simulink model "Acq_HDL"  (R2019b)
settings: Solver=VariableStepAuto  StartTime=0.0  StopTime=time  RelTol=1e-3
values from neighbouring files (symbols this model uses):
  fs = 16367600    [config.m]
  Len = ceil(ms*fs/1000)    [config.m]
libraries: commseqgen3 x4, simulink x3, dsphdlxfrm x2, hdlsllib x2, dspsigops x2, dspswit3 x1, dspsrcs4 x1
settings Model: Creator=nishantmittal  LastModifiedBy=nishantmittal

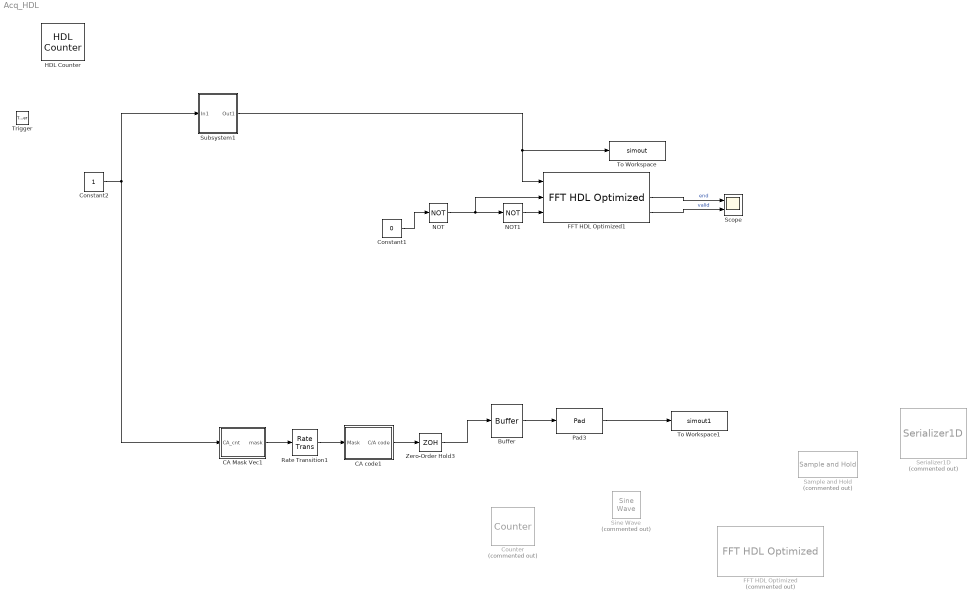
== system Acq_HDL ==
  Trigger : TriggerPort  VariantControl=Variant  PortDimensions=1
  Buffer : Buffer  N=Len  OutputFrames=off
  CA Mask Vec1 : MATLAB Function  TreatAsAtomicUnit=on
  CA code1 : Subsystem
  Constant1 : Constant  Value=0  OutDataTypeStr=Inherit: Inherit via back propagation  SampleTime=-1
  Constant2 : Constant  OutDataTypeStr=Inherit: Inherit via back propagation  SampleTime=-1
  Counter : dspswit3/Counter  Commented=on  Direction=Up  CountEvent=Rising edge  CounterSize=User defined  MaxCount=Len  InitialCount=1  Output=Count and Hit  HitValue=Len  ResetInput=on  SamplesPerFrame=1  Ts=1  CntDtype=single  HitDtype=Logical
  FFT HDL Optimized : dsphdlxfrm/FFT HDL Optimized  Commented=on  FFTLength=2^nextpow2(Len)  Architecture=Streaming Radix 2^2  ComplexMultiplication=Use 4 multipliers and 2 adders  BitReversedOutput=on  BitReversedInput=off  Normalize=off  SimulateUsing=Code generation  RoundingMethod=Floor  ResetInputPort=on  StartOutputPort=off  EndOutputPort=on
      settings: SourceProductName=DSP System Toolbox  SourceProductBaseCode=DS
  FFT HDL Optimized1 : dsphdlxfrm/FFT HDL Optimized  FFTLength=64  Architecture=Streaming Radix 2^2  ComplexMultiplication=Use 4 multipliers and 2 adders  BitReversedOutput=on  BitReversedInput=off  Normalize=off  SimulateUsing=Code generation  RoundingMethod=Floor  ResetInputPort=on  StartOutputPort=off  EndOutputPort=on
      settings: SourceProductName=DSP System Toolbox  SourceProductBaseCode=DS
  HDL Counter : hdlsllib/Sources/HDL Counter  CountType=Count limited  CountInit=0  CountStep=1  CountMax=25  CountFromType=Initial value  CountFrom=0  CountResetPort=off  CountLoadPort=off  CountEnbPort=off  CountDirPort=off  CountDataType=Unsigned  CountWordLen=8  CountFracLen=0  CountSampTime=1
      settings: SourceProductName=Simulink
  NOT : Logic  Operator=NOT  IconShape=distinctive  AllPortsSameDT=off  OutDataTypeStr=boolean
  NOT1 : Logic  Operator=NOT  IconShape=distinctive  AllPortsSameDT=off  OutDataTypeStr=boolean
  Pad3 : dspsigops/Pad  padAlong=Columns  dimsToPad=1  valSrc=Specify via dialog  padVal=0  spec=Output size  padNumOutRowsSpecMethod=Next power of two  numOutRows=1  padNumOutColsSpecMethod=Next power of two  numOutCols=1  isVarDimsMode=off  padBeginning=0  padEnd=0  outSizeMode=User-specified  outSize=1  padSigAt=End  trunc_flag=None  roundingMode=Floor  overflowMode=off  truncOrWrapMode=Truncate  wrap_flag=None
      settings: SourceProductName=DSP System Toolbox  SourceProductBaseCode=DS
  Rate Transition1 : RateTransition  Deterministic=off  OutPortSampleTime=1/(1.023e6)
  Sample and Hold : dspsigops/Sample and Hold  Commented=on  trig=Rising edge  initCond=0  latchinput=on
  Scope : Scope  NumInputPorts=2
  Serializer1D : hdlsllib/HDL Operations/Serializer1D  Commented=on  Ratio=1  IdleCycles=0  validIn=on  startOut=on  validOut=on  inputDataDimensions=-1  inputSampleTime=-1  inputSignalType=auto
      settings: SourceProductName=Simulink  SourceProductBaseCode=SL
  Sine Wave : dspsrcs4/Sine Wave  Commented=on  Amplitude=1  Frequency=100  Phase=0  SampleMode=Discrete  OutComplex=Real  CompMethod=Trigonometric fcn  TableSize=Speed  SampleTime=1/1000  SamplesPerFrame=1  ResetState=Restart at time zero  OutputFrames=off  dataType=single  wordLen=16  udDataType=sfix(16)  fracBitsMode=Best precision  numFracBits=15  OutDataTypeStr=single  LastOutDataTypeStr=single
  Subsystem1 : Subsystem
  To Workspace : ToWorkspace  VariableName=simout  SaveFormat=Timeseries  SampleTime=-1
  To Workspace1 : ToWorkspace  VariableName=simout1  SaveFormat=Timeseries  SampleTime=-1
  Zero-Order Hold3 : ZeroOrderHold  SampleTime=1/fs
  wires:
  Constant1/1 -> NOT/1
  NOT/1 -> FFT HDL Optimized1/2, NOT1/1
  NOT1/1 -> FFT HDL Optimized1/3
  FFT HDL Optimized1/2 -> Scope/1  "end"
  FFT HDL Optimized1/3 -> Scope/2  "valid"
  Zero-Order Hold3/1 -> Buffer/1
  Rate Transition1/1 -> CA code1/1(Mask)
  Constant2/1 -> Subsystem1/1(In1), CA Mask Vec1/1(CA_cnt)
  CA Mask Vec1/1(mask) -> Rate Transition1/1
  CA code1/1(C/A code) -> Zero-Order Hold3/1
  Buffer/1 -> Pad3/1
  Pad3/1 -> To Workspace1/1
  Subsystem1/1(Out1) -> To Workspace/1, FFT HDL Optimized1/1

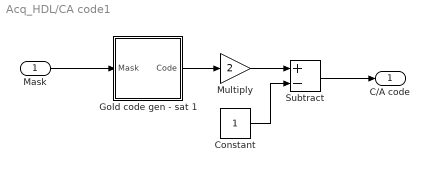
== system Acq_HDL/CA code1 ==
  Mask : Inport
  Constant : Constant
  Gold code gen - sat 1 : Subsystem
  Multiply : Gain  Gain=2
  Subtract : Sum  Inputs=+-
  C/A code : Outport
  wires:
  Subtract/1 -> C/A code/1
  Multiply/1 -> Subtract/1
  Gold code gen - sat 1/1(Code) -> Multiply/1
  Constant/1 -> Subtract/2
  Mask/1 -> Gold code gen - sat 1/1(Mask)

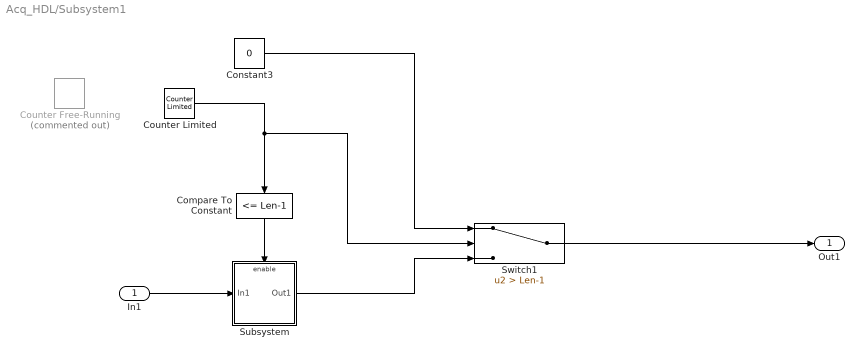
== system Acq_HDL/Subsystem1 ==
  In1 : Inport
  Compare To Constant : simulink/Logic and Bit Operations/Compare To Constant  relop=<=  const=Len-1  OutDataTypeStr=boolean
  Constant3 : Constant  Value=0  OutDataTypeStr=Inherit: Inherit via back propagation  SampleTime=-1
  Counter Free-Running : simulink/Sources/Counter Free-Running  Commented=on  NumBits=3+ nextpow2(Len)  tsamp=-1
  Counter Limited : simulink/Sources/Counter Limited  uplimit=2^nextpow2(Len) - 1  tsamp=-1
  Subsystem : Subsystem
  Switch1 : Switch  Criteria=u2 > Threshold  Threshold=Len-1
  Out1 : Outport
  wires:
  Subsystem/1(Out1) -> Switch1/3
  Switch1/1 -> Out1/1
  In1/1 -> Subsystem/1(In1)
  Compare To Constant/1 -> Subsystem/Enable
  Constant3/1 -> Switch1/1
  Counter Limited/1 -> Switch1/2, Compare To Constant/1

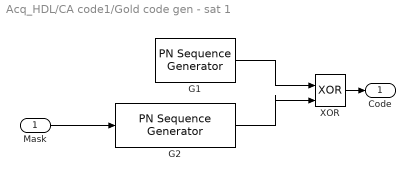
== system Acq_HDL/CA code1/Gold code gen - sat 1 ==
  Mask : Inport
  G1 : commseqgen3/PN Sequence Generator  poly=[10 7 0]  ini_sta=[1 1 1 1 1 1 1 1 1 1]  outBitMaskSource=Dialog parameter  shift=[0 0 0 0 0 0 0 0 0 1]  outVarSiz=off  maxOutSizeMode=Dialog parameter  maxOutSize=[10 1]  Ts=1/(1.023e6)  sampPerFrame=1  reset=off  bitPackedOutputs=off  outDataType=boolean  numPackedBits=8  bitPackDataSigned=off  bitPackedOutDType=double
      settings: SourceProductName=Communications Toolbox
  G2 : commseqgen3/PN Sequence Generator  poly=[10 8 7 4 2 1 0]  ini_sta=[1 1 1 1 1 1 1 1 1 1]  outBitMaskSource=Input port  shift=[0 1 0 0 0 1 0 0 0 0]  outVarSiz=off  maxOutSizeMode=Dialog parameter  maxOutSize=[10 1]  Ts=1/(1.023e6)  sampPerFrame=1  reset=off  bitPackedOutputs=off  outDataType=boolean  numPackedBits=8  bitPackDataSigned=off  bitPackedOutDType=double
      settings: SourceProductName=Communications Toolbox
  XOR : Logic  Operator=XOR  IconShape=distinctive  AllPortsSameDT=off  OutDataTypeStr=boolean
  Code : Outport
  wires:
  G2/1 -> XOR/2
  XOR/1 -> Code/1
  G1/1 -> XOR/1
  Mask/1 -> G2/1

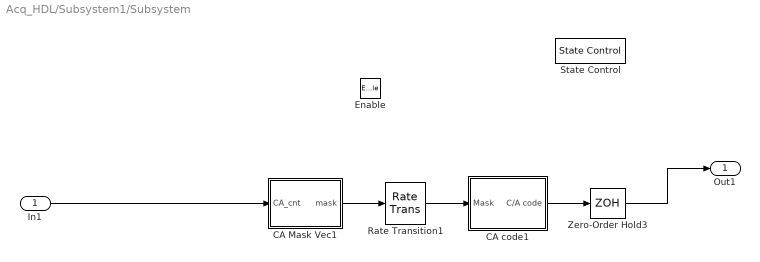
== system Acq_HDL/Subsystem1/Subsystem ==
  In1 : Inport
  Enable : EnablePort
  CA Mask Vec1 : MATLAB Function  TreatAsAtomicUnit=on
  CA code1 : Subsystem
  Rate Transition1 : RateTransition  Deterministic=off  OutPortSampleTime=1/(1.023e6)
  State Control : StateControl
  Zero-Order Hold3 : ZeroOrderHold  SampleTime=1/fs
  Out1 : Outport
  wires:
  Zero-Order Hold3/1 -> Out1/1
  In1/1 -> CA Mask Vec1/1(CA_cnt)
  Rate Transition1/1 -> CA code1/1(Mask)
  CA Mask Vec1/1(mask) -> Rate Transition1/1
  CA code1/1(C/A code) -> Zero-Order Hold3/1

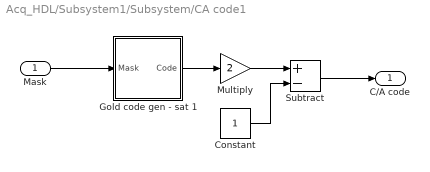
== system Acq_HDL/Subsystem1/Subsystem/CA code1 ==
  Mask : Inport
  Constant : Constant
  Gold code gen - sat 1 : Subsystem
  Multiply : Gain  Gain=2
  Subtract : Sum  Inputs=+-
  C/A code : Outport
  wires:
  Subtract/1 -> C/A code/1
  Multiply/1 -> Subtract/1
  Gold code gen - sat 1/1(Code) -> Multiply/1
  Constant/1 -> Subtract/2
  Mask/1 -> Gold code gen - sat 1/1(Mask)

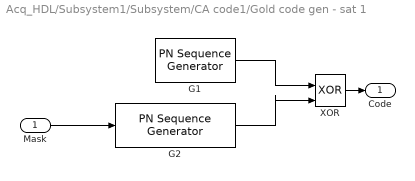
== system Acq_HDL/Subsystem1/Subsystem/CA code1/Gold code gen - sat 1 ==
  Mask : Inport
  G1 : commseqgen3/PN Sequence Generator  poly=[10 7 0]  ini_sta=[1 1 1 1 1 1 1 1 1 1]  outBitMaskSource=Dialog parameter  shift=[0 0 0 0 0 0 0 0 0 1]  outVarSiz=off  maxOutSizeMode=Dialog parameter  maxOutSize=[10 1]  Ts=1/(1.023e6)  sampPerFrame=1  reset=off  bitPackedOutputs=off  outDataType=boolean  numPackedBits=8  bitPackDataSigned=off  bitPackedOutDType=double
      settings: SourceProductName=Communications Toolbox
  G2 : commseqgen3/PN Sequence Generator  poly=[10 8 7 4 2 1 0]  ini_sta=[1 1 1 1 1 1 1 1 1 1]  outBitMaskSource=Input port  shift=[0 1 0 0 0 1 0 0 0 0]  outVarSiz=off  maxOutSizeMode=Dialog parameter  maxOutSize=[10 1]  Ts=1/(1.023e6)  sampPerFrame=1  reset=off  bitPackedOutputs=off  outDataType=boolean  numPackedBits=8  bitPackDataSigned=off  bitPackedOutDType=double
      settings: SourceProductName=Communications Toolbox
  XOR : Logic  Operator=XOR  IconShape=distinctive  AllPortsSameDT=off  OutDataTypeStr=boolean
  Code : Outport
  wires:
  G2/1 -> XOR/2
  XOR/1 -> Code/1
  G1/1 -> XOR/1
  Mask/1 -> G2/1

== matlab function Acq_HDL/CA Mask Vec1 ==
  data: CA_cnt input; mask output
function mask = fcn(CA_cnt)

phase = [2 6; 3 7; 4 8; 5 9; 1 9; 2 10; 1 8; 2 9; 3 10; 2 3; 3 4; 5 6; 6 7; 7 8; 8 9; 9 10; 1 4; 2 5; 3 6; 4 7; 5 8; 6 9; 1 3; 4 6; 5 7; 6 8; 7 9; 8 10; 1 6; 2 7; 3 8; 4 9];
mask_points = phase(CA_cnt, :);
mask = zeros(1,10);
mask(mask_points) = 1;

== matlab function Acq_HDL/Subsystem1/Subsystem/CA Mask Vec1 ==
  data: CA_cnt input; mask output
function mask = fcn(CA_cnt)

phase = [2 6; 3 7; 4 8; 5 9; 1 9; 2 10; 1 8; 2 9; 3 10; 2 3; 3 4; 5 6; 6 7; 7 8; 8 9; 9 10; 1 4; 2 5; 3 6; 4 7; 5 8; 6 9; 1 3; 4 6; 5 7; 6 8; 7 9; 8 10; 1 6; 2 7; 3 8; 4 9];
mask_points = phase(CA_cnt, :);
mask = zeros(1,10);
mask(mask_points) = 1;
